simulink model "full_observer_2"  (R2020b)
settings: Solver=FixedStepAuto  StartTime=0.0  StopTime=15  FixedStep=0.01  RelTol=1e-3
values from neighbouring files (symbols this model uses):
  G = -J_RH*(M_M*L/2+M*l)*(J_RH+N^2*J_m+j)*g    (= -0.22537747671)    [aaaaaaaaaaaaaaaaaaaaaaaaa.m]    (also in disturb_estimation.m = -0.0465293382657; full_obs2.m = -0.0465293382657; fuulll_feedback.m = -0.0465293382657; reduced_observre_2.m = -0.0465293382657)
  H = -N*K_m*J_RH    (= -0.00759948)    [aaaaaaaaaaaaaaaaaaaaaaaaa.m]    (also in disturb_estimation.m = -0.00486576; full_obs2.m = -0.00486576; fuulll_feedback.m = -0.00486576; reduced_observre_2.m = -0.00486576)
  k1 = K(1)    [disturb_estimation.m]    (also in full_obs2.m; fuulll_feedback.m; reduced_observre_2.m)
  k2 = K(2)    [disturb_estimation.m]    (also in full_obs2.m; fuulll_feedback.m; reduced_observre_2.m)
  k3 = K(3)    [disturb_estimation.m]    (also in full_obs2.m; fuulll_feedback.m; reduced_observre_2.m)
  k4 = K(4)    [disturb_estimation.m]    (also in full_obs2.m; fuulll_feedback.m; reduced_observre_2.m)
  k5 = K(5)    [disturb_estimation.m]    (also in full_obs2.m; fuulll_feedback.m; reduced_observre_2.m)
  K_m = 0.0109    [aaaaaaaaaaaaaaaaaaaaaaaaa.m]    (also in disturb_estimation.m; full_obs2.m; fuulll_feedback.m; reduced_observre_2.m)
  l1 = L(1)    [disturb_estimation.m]    (also in full (2).m = 0.06; full_obs2.m)
  l2 = L(2)    [disturb_estimation.m]    (also in full (2).m = 0.6329; full_obs2.m)
  l3 = L(3)    [disturb_estimation.m]    (also in full (2).m = 0.3; full_obs2.m)
  l4 = L(4)    [disturb_estimation.m]    (also in full (2).m = 0.0875; full_obs2.m)
  l5 = L(5)    [disturb_estimation.m]    (also in full (2).m = 0.0254; full_obs2.m)
  L_m = 0.145    [aaaaaaaaaaaaaaaaaaaaaaaaa.m]    (also in disturb_estimation.m; full_obs2.m; fuulll_feedback.m; reduced_observre_2.m)
  N = 14    [aaaaaaaaaaaaaaaaaaaaaaaaa.m]    (also in disturb_estimation.m = 3; full (2).m = -1.06605676; full_obs2.m = 3; fuulll_feedback.m = 3)
  R_m = 1.6    [aaaaaaaaaaaaaaaaaaaaaaaaa.m]    (also in disturb_estimation.m; full_obs2.m; fuulll_feedback.m; reduced_observre_2.m)
  T = (M_M*L/2+M*l)*(J_RH+N^2*J_m+j)*g    (= 4.52565214276)    [aaaaaaaaaaaaaaaaaaaaaaaaa.m]    (also in disturb_estimation.m = 0.312697165764; full (2).m = [T1;T2;T3;T4;T5;T6;T7]; full_obs2.m = 0.312697165764; fuulll_feedback.m = 0.312697165764)
  W = (J_M+M*l^2)*(J_RH+N^2*J_m+j)-(J_RH)^2    (= 0.0397505665657)    [aaaaaaaaaaaaaaaaaaaaaaaaa.m]    (also in disturb_estimation.m = -0.0192235420783; full (2).m = blkdiag(W_1,W_2,W_3,W_4,W_5,W_6,W_7); full_obs2.m = -0.0192235420783; fuulll_feedback.m = -0.0192235420783)
  Z = (J_M+M*l^2)*(J_RH+N^2*J_m+j)^2-J_RH^2*(J_RH+N^2*J_m+j)    (= 0.251295170273)    [aaaaaaaaaaaaaaaaaaaaaaaaa.m]    (also in disturb_estimation.m = -0.00839686182665; full_obs2.m = -0.00839686182665; fuulll_feedback.m = -0.00839686182665; reduced_observre_2.m = -0.00839686182665)
settings Model: Creator=A family  LastModifiedBy=A family

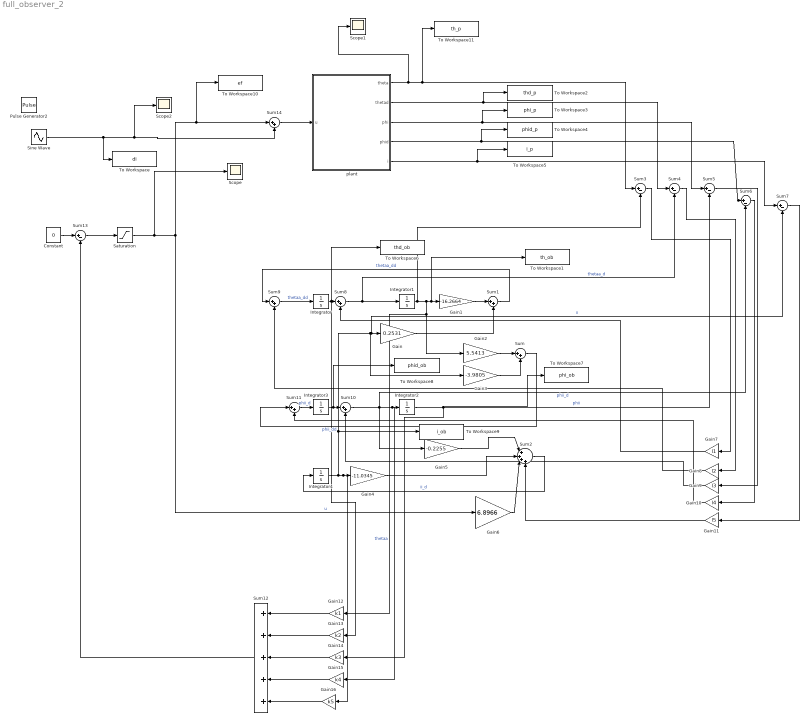
== system full_observer_2 ==
  Constant : Constant  Value=0
  Gain : Gain  Gain=0.2531
  Gain1 : Gain  Gain=-16.2664
  Gain10 : Gain  Gain=l4
  Gain11 : Gain  Gain=l5
  Gain12 : Gain  Gain=k1
  Gain13 : Gain  Gain=k2
  Gain14 : Gain  Gain=k3
  Gain15 : Gain  Gain=k4
  Gain16 : Gain  Gain=k5
  Gain2 : Gain  Gain=5.5413
  Gain3 : Gain  Gain=-3.9805
  Gain4 : Gain  Gain=-11.0345
  Gain5 : Gain  Gain=-0.2255
  Gain6 : Gain  Gain=6.8966
  Gain7 : Gain  Gain=l1
  Gain8 : Gain  Gain=l2
  Gain9 : Gain  Gain=l3
  Integrator{,1..4} (5 alike) : Integrator
  Pulse Generator2 : DiscretePulseGenerator  PulseType=Time based  Amplitude=10  Period=5  PulseWidth=5
  Saturation : Saturate  UpperLimit=6  LowerLimit=-6
  Scope : Scope
  Scope1 : Scope
  Scope2 : Scope
  Sine Wave : Sin  Amplitude=1.5  SampleTime=0
  Sum{,1,8..11,14} (7 alike) : Sum  Inputs=|++
  Sum12 : Sum  Inputs=+++++
  Sum{3..7,13} (6 alike) : Sum  Inputs=|+-
  Sum2 : Sum  Inputs=|++++
  To Workspace : ToWorkspace  VariableName=di  SampleTime=-1
  To Workspace1 : ToWorkspace  VariableName=th_ob  SampleTime=-1
  To Workspace10 : ToWorkspace  VariableName=ef  SampleTime=-1
  To Workspace11 : ToWorkspace  VariableName=th_p  SampleTime=-1
  To Workspace2 : ToWorkspace  VariableName=thd_p  SampleTime=-1
  To Workspace3 : ToWorkspace  VariableName=phi_p  SampleTime=-1
  To Workspace4 : ToWorkspace  VariableName=phid_p  SampleTime=-1
  To Workspace5 : ToWorkspace  VariableName=i_p  SampleTime=-1
  To Workspace6 : ToWorkspace  VariableName=thd_ob  SampleTime=-1
  To Workspace7 : ToWorkspace  VariableName=phi_ob  SampleTime=-1
  To Workspace8 : ToWorkspace  VariableName=phid_ob  SampleTime=-1
  To Workspace9 : ToWorkspace  VariableName=i_ob  SampleTime=-1
  plant : Subsystem
  wires:
  Sum8/1 -> Sum4/2, Integrator1/1  "thetaa_d"
  Integrator1/1 -> Gain12/1, Gain2/1, To Workspace1/1, Gain1/1, Sum3/2  "thetaa"
  Sum1/1 -> Sum9/1  "thetaa_dd"
  Gain/1 -> Sum1/2
  Gain1/1 -> Sum1/1
  Sum/1 -> Sum11/1  "phii_dd"
  Sum10/1 -> Gain15/1, Integrator2/1, Sum6/2, Gain5/1  "phii_d"
  Integrator2/1 -> Gain14/1, To Workspace7/1, Sum5/2  "phii"
  Integrator4/1 -> Gain16/1, Gain4/1, To Workspace9/1, Sum7/2, Gain/1, Gain3/1  "ii"
  Gain2/1 -> Sum/1
  Gain3/1 -> Sum/2
  Sum2/1 -> Integrator4/1  "ii_d"
  Gain4/1 -> Sum2/2
  Gain5/1 -> Sum2/1
  Saturation/1 -> Scope/1, To Workspace10/1, Sum14/1, Gain6/1  "u"
  Gain6/1 -> Sum2/3
  plant/5(i) -> To Workspace5/1, Sum7/1
  plant/3(phi) -> To Workspace3/1, Sum5/1
  plant/4(phid) -> To Workspace4/1, Sum6/1
  plant/2(thetad) -> To Workspace2/1, Sum4/1
  plant/1(theta) -> Scope1/1, To Workspace11/1, Sum3/1
  Sum3/1 -> Gain7/1
  Sum4/1 -> Gain8/1
  Sum5/1 -> Gain9/1
  Sum6/1 -> Gain10/1
  Sum7/1 -> Gain11/1
  Integrator/1 -> Gain13/1, To Workspace6/1, Sum8/1
  Gain7/1 -> Sum8/2
  Gain8/1 -> Sum9/2
  Sum9/1 -> Integrator/1  "thetaa_dd"
  Gain9/1 -> Sum10/2
  Sum11/1 -> Integrator3/1  "phii_d"
  Gain10/1 -> Sum11/2
  Gain11/1 -> Sum2/4
  Integrator3/1 -> To Workspace8/1, Sum10/1
  Gain15/1 -> Sum12/4
  Sum12/1 -> Sum13/2
  Gain14/1 -> Sum12/3
  Gain13/1 -> Sum12/2
  Gain12/1 -> Sum12/1
  Gain16/1 -> Sum12/5
  Sum13/1 -> Saturation/1
  Constant/1 -> Sum13/1
  Sine Wave/1 -> To Workspace/1, Scope2/1, Sum14/2
  Sum14/1 -> plant/1(u)

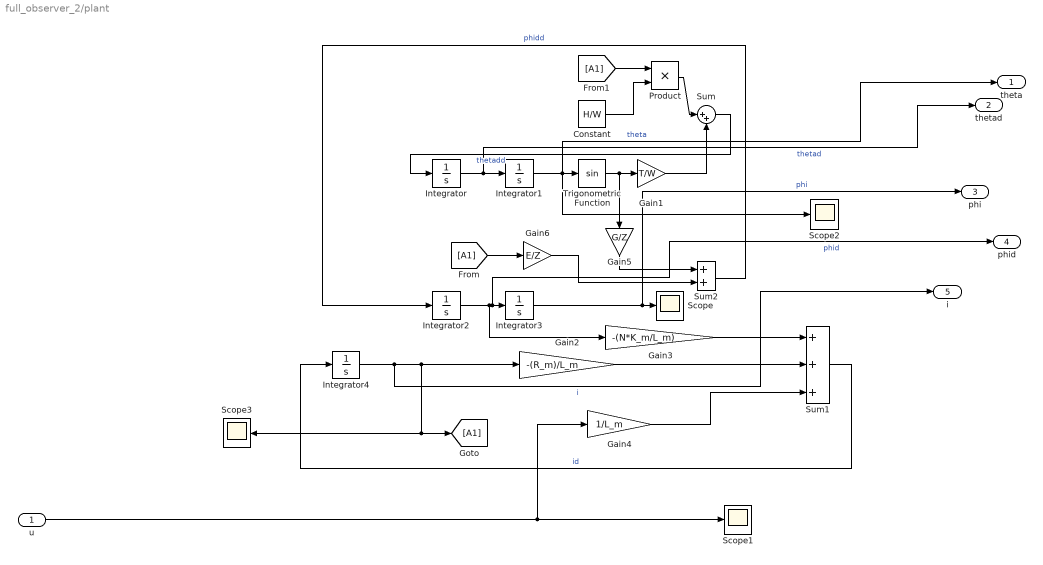
== system full_observer_2/plant ==
  u : Inport
  Constant : Constant  Value=H/W
  Gain1 : Gain  Gain=T/W
  Gain2 : Gain  Gain=-(R_m)/L_m
  Gain3 : Gain  Gain=-(N*K_m/L_m)
  Gain4 : Gain  Gain=1/L_m
  Gain5 : Gain  Gain=G/Z
  Gain6 : Gain  Gain=E/Z
  Integrator{,2..4} (4 alike) : Integrator
  Integrator1 : Integrator  InitialCondition=20*pi/180
  Product : Product
  Scope{,1..3} (4 alike) : Scope
  Sum : Sum  Inputs=|++
  Sum1 : Sum  Inputs=+++
  Sum2 : Sum
  Trigonometric Function : Trigonometry
  theta : Outport
  thetad : Outport  Port=2
  phi : Outport  Port=3
  phid : Outport  Port=4
  i : Outport  Port=5
  wires:
  Integrator/1 -> thetad/1, Integrator1/1  "thetad"
  Integrator2/1 -> phid/1, Integrator3/1, Gain3/1  "phid"
  Integrator4/1 -> Gain2/1, Scope3/1, [A1], i/1  "i"
  Gain5/1 -> Sum2/1
  u/1 -> Scope1/1, Gain4/1
  Product/1 -> Sum/1
  Sum2/1 -> Integrator2/1  "phidd"
  Integrator1/1 -> Scope2/1, theta/1, Trigonometric Function/1  "theta"
  Gain4/1 -> Sum1/3
  Integrator3/1 -> phi/1, Scope/1  "phi"
  [A1] -> Gain6/1
  Gain6/1 -> Sum2/2
  [A1] -> Product/1
  Constant/1 -> Product/2
  Gain1/1 -> Sum/2
  Trigonometric Function/1 -> Gain5/1, Gain1/1
  Gain3/1 -> Sum1/1
  Gain2/1 -> Sum1/2
  Sum1/1 -> Integrator4/1  "id"
  Sum/1 -> Integrator/1  "thetadd"
